simulink model "Q1"  (R2020b)
settings: Solver=VariableStepAuto  StartTime=0.0  StopTime=30  RelTol=1e-3
undefined symbols (not defined in the file): A_num, B_num, C_num, K_fast, K_slow
settings Model: Creator=asus  LastModifiedBy=asus

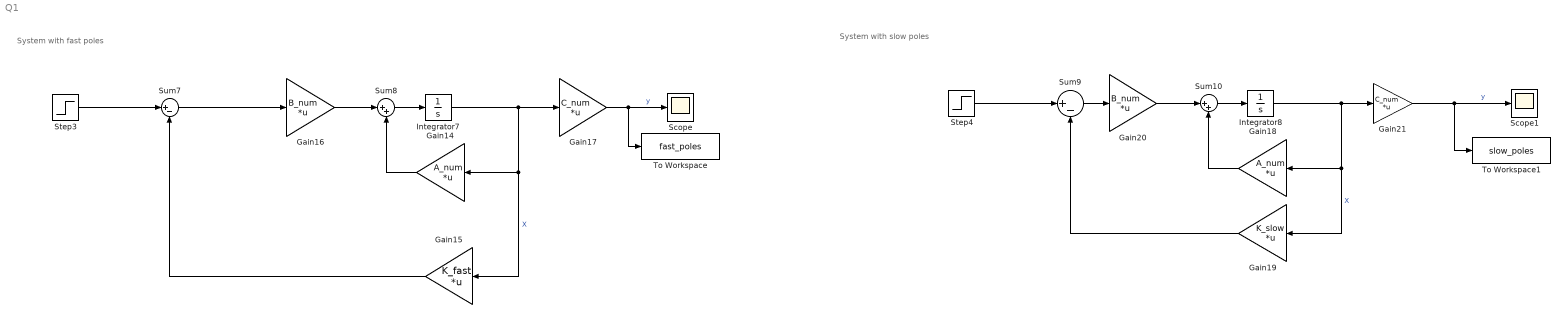
== system Q1 ==
  note: System with slow poles
  note: System with fast poles
  Gain14 : Gain  Gain=A_num  Multiplication=Matrix(K*u)
  Gain15 : Gain  Gain=K_fast  Multiplication=Matrix(K*u)
  Gain16 : Gain  Gain=B_num  Multiplication=Matrix(K*u)
  Gain17 : Gain  Gain=C_num  Multiplication=Matrix(K*u)
  Gain18 : Gain  Gain=A_num  Multiplication=Matrix(K*u)
  Gain19 : Gain  Gain=K_slow  Multiplication=Matrix(K*u)
  Gain20 : Gain  Gain=B_num  Multiplication=Matrix(K*u)
  Gain21 : Gain  Gain=C_num  Multiplication=Matrix(K*u)
  Integrator7 : Integrator
  Integrator8 : Integrator
  Scope : Scope
  Scope1 : Scope
  Step3 : Step  SampleTime=0
  Step4 : Step  SampleTime=0
  Sum10 : Sum  Inputs=|++
  Sum7 : Sum  Inputs=|+-
  Sum8 : Sum  Inputs=|++
  Sum9 : Sum  Inputs=|+-
  To Workspace : ToWorkspace  VariableName=fast_poles  SaveFormat=Timeseries  SampleTime=-1
  To Workspace1 : ToWorkspace  VariableName=slow_poles  SaveFormat=Timeseries  SampleTime=-1
  wires:
  Gain21/1 -> To Workspace1/1, Scope1/1  "y"
  Gain15/1 -> Sum7/2
  Step4/1 -> Sum9/1
  Sum10/1 -> Integrator8/1
  Integrator7/1 -> Gain17/1, Gain15/1, Gain14/1  "X"
  Sum7/1 -> Gain16/1
  Gain18/1 -> Sum10/2
  Integrator8/1 -> Gain19/1, Gain18/1, Gain21/1  "X"
  Sum8/1 -> Integrator7/1
  Gain16/1 -> Sum8/1
  Sum9/1 -> Gain20/1
  Gain20/1 -> Sum10/1
  Gain14/1 -> Sum8/2
  Gain17/1 -> To Workspace/1, Scope/1  "y"
  Gain19/1 -> Sum9/2
  Step3/1 -> Sum7/1
